simulink model "sanz2016_simu"  (R2023a)
settings: Solver=VariableStepAuto  StartTime=0.0  StopTime=Tsim  RelTol=1e-3
values from neighbouring files (symbols this model uses):
  A = [0 1; -9 3]    [sanz2016_code.m]
  Aw1 = AH_w1    [sanz2016_code.m]
  Aw2 = AH_w2    [sanz2016_code.m]
  B = [0 1]'    [sanz2016_code.m]
  B1w1 = AH_w1*BH_w1*pinv(B)-BH_w1*pinv(B)*A    [sanz2016_code.m]
  B1w2 = AH_w2*BH_w2*pinv(B)-BH_w2*pinv(B)*A    [sanz2016_code.m]
  B2w1 = BH_w1    [sanz2016_code.m]
  B2w2 = BH_w2    [sanz2016_code.m]
  C1 = CH    [sanz2016_code.m]
  C2w1 = CH*BH_w1*pinv(B)    [sanz2016_code.m]
  C2w2 = CH*BH_w2*pinv(B)    [sanz2016_code.m]
  h = 0.5    [sanz2016_code.m]
  K = [-45 -18]    [sanz2016_code.m]
  N = 500    [sanz2016_code.m]
  x0 = [1.5; 1]    [sanz2016_code.m]
undefined symbols (not defined in the file or in its folder): Ad, Bd, Cd, Dd, KSoma, Q, tal
settings Model: Creator=Vasco  LastModifiedBy=Vasco
settings DataIOCC: ReturnWorkspaceOutputs=off

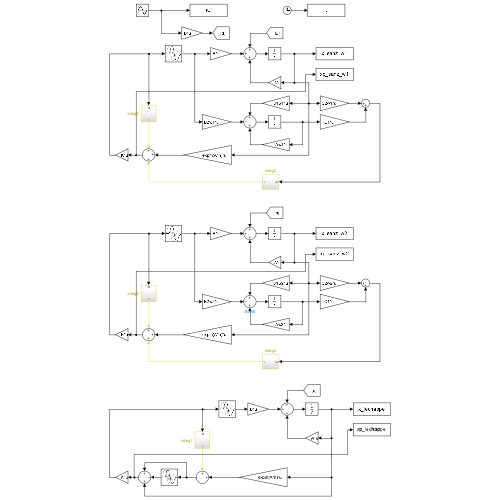
[thumbnail: Simulink's stored preview of the top-level diagram]
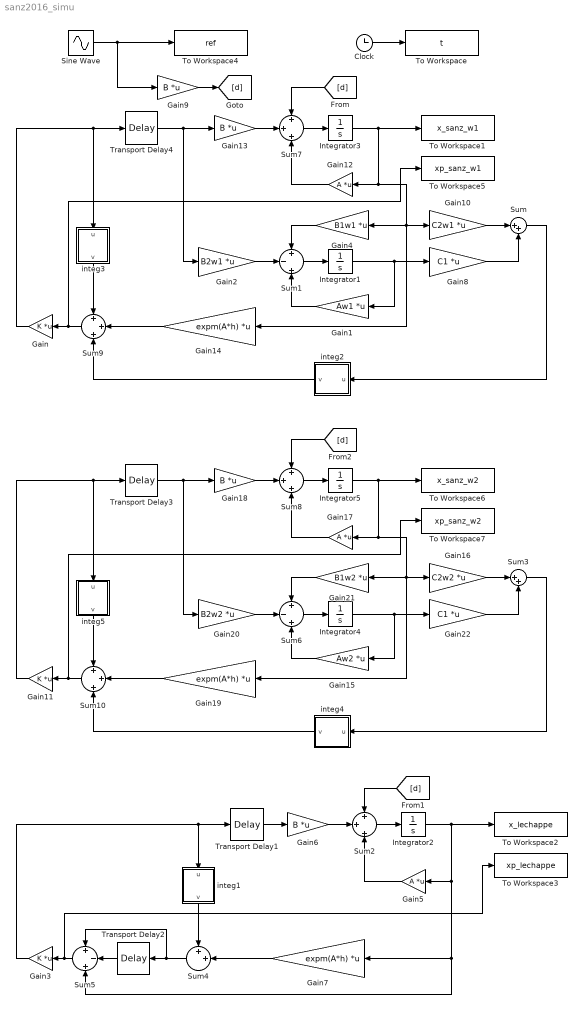
== system sanz2016_simu ==
  Clock : Clock
  Gain : Gain  Gain=K  Multiplication=Matrix(K*u)
  Gain1 : Gain  Gain=Aw1  Multiplication=Matrix(K*u)
  Gain10 : Gain  Gain=C2w1  Multiplication=Matrix(K*u)
  Gain11 : Gain  Gain=K  Multiplication=Matrix(K*u)
  Gain12 : Gain  Gain=A  Multiplication=Matrix(K*u)
  Gain{6,9,13,18} (4 alike) : Gain  Gain=B  Multiplication=Matrix(K*u)
  Gain14 : Gain  Gain=expm(A*h)  Multiplication=Matrix(K*u)
  Gain15 : Gain  Gain=Aw2  Multiplication=Matrix(K*u)
  Gain16 : Gain  Gain=C2w2  Multiplication=Matrix(K*u)
  Gain17 : Gain  Gain=A  Multiplication=Matrix(K*u)
  Gain19 : Gain  Gain=expm(A*h)  Multiplication=Matrix(K*u)
  Gain2 : Gain  Gain=B2w1  Multiplication=Matrix(K*u)
  Gain20 : Gain  Gain=B2w2  Multiplication=Matrix(K*u)
  Gain21 : Gain  Gain=B1w2  Multiplication=Matrix(K*u)
  Gain22 : Gain  Gain=C1  Multiplication=Matrix(K*u)
  Gain3 : Gain  Gain=K  Multiplication=Matrix(K*u)
  Gain4 : Gain  Gain=B1w1  Multiplication=Matrix(K*u)
  Gain5 : Gain  Gain=A  Multiplication=Matrix(K*u)
  Gain7 : Gain  Gain=expm(A*h)  Multiplication=Matrix(K*u)
  Gain8 : Gain  Gain=C1  Multiplication=Matrix(K*u)
  Integrator1 : Integrator
  Integrator2 : Integrator  InitialCondition=x0
  Integrator3 : Integrator  InitialCondition=x0
  Integrator4 : Integrator
  Integrator5 : Integrator  InitialCondition=x0
  Sine Wave : Sin  Amplitude=3  Frequency=0.5  SampleTime=0
  Sum : Sum  Inputs=|++
  Sum1 : Sum  Inputs=+|-|+
  Sum{2,7..10} (5 alike) : Sum  Inputs=+|+|+
  Sum3 : Sum  Inputs=|++
  Sum4 : Sum  Inputs=++|
  Sum5 : Sum  Inputs=+|-|+
  Sum6 : Sum  Inputs=+|-|+
  To Workspace : ToWorkspace  VariableName=t  SampleTime=-1
  To Workspace1 : ToWorkspace  VariableName=x_sanz_w1  SampleTime=-1
  To Workspace2 : ToWorkspace  VariableName=x_lechappe  SampleTime=-1
  To Workspace3 : ToWorkspace  VariableName=xp_lechappe  SampleTime=-1
  To Workspace4 : ToWorkspace  VariableName=ref  SampleTime=-1
  To Workspace5 : ToWorkspace  VariableName=xp_sanz_w1  SampleTime=-1
  To Workspace6 : ToWorkspace  VariableName=x_sanz_w2  SampleTime=-1
  To Workspace7 : ToWorkspace  VariableName=xp_sanz_w2  SampleTime=-1
  Transport Delay{1..4} (4 alike) : TransportDelay  DelayTime=h
  integ1 : Subsystem
  integ2 : Subsystem
  integ3 : Subsystem
  integ4 : Subsystem
  integ5 : Subsystem
  wires:
  Clock/1 -> To Workspace/1
  integ3/1(v) -> Sum9/1
  Gain13/1 -> Sum7/2
  Gain12/1 -> Sum7/3
  Sum7/1 -> Integrator3/1
  Transport Delay4/1 -> Gain13/1, Gain2/1
  Gain14/1 -> Sum9/2
  Gain5/1 -> Sum2/3
  integ1/1(v) -> Sum4/1
  Sum2/1 -> Integrator2/1
  Gain7/1 -> Sum4/2
  Gain6/1 -> Sum2/2
  Transport Delay1/1 -> Gain6/1
  Sum5/1 -> Gain3/1, To Workspace3/1
  Sum4/1 -> Transport Delay2/1, Sum5/1
  Transport Delay2/1 -> Sum5/2
  Sine Wave/1 -> Gain9/1, To Workspace4/1
  Sum9/1 -> To Workspace5/1, Gain/1
  Gain3/1 -> integ1/1(u), Transport Delay1/1
  Gain/1 -> Transport Delay4/1, integ3/1(u)
  Integrator2/1 -> Sum5/3, Gain7/1, Gain5/1, To Workspace2/1
  Gain2/1 -> Sum1/2
  Gain4/1 -> Sum1/1
  Gain1/1 -> Sum1/3
  Integrator1/1 -> Gain8/1, Gain1/1
  Integrator3/1 -> Gain10/1, Gain4/1, Gain14/1, Gain12/1, To Workspace1/1
  Sum1/1 -> Integrator1/1
  Gain10/1 -> Sum/1
  Gain8/1 -> Sum/2
  Sum/1 -> integ2/1(u)
  integ2/1(v) -> Sum9/3
  Gain9/1 -> [d]
  [d] -> Sum7/1
  [d] -> Sum2/1
  integ4/1(v) -> Sum10/3
  Gain16/1 -> Sum3/1
  Gain21/1 -> Sum6/1
  Gain15/1 -> Sum6/3
  Gain11/1 -> Transport Delay3/1, integ5/1(u)
  Sum10/1 -> To Workspace7/1, Gain11/1
  Gain18/1 -> Sum8/2
  Gain17/1 -> Sum8/3
  Integrator4/1 -> Gain22/1, Gain15/1
  Integrator5/1 -> Gain16/1, Gain21/1, Gain19/1, Gain17/1, To Workspace6/1
  Gain22/1 -> Sum3/2
  Gain19/1 -> Sum10/2
  Sum8/1 -> Integrator5/1
  integ5/1(v) -> Sum10/1
  Sum6/1 -> Integrator4/1
  Transport Delay3/1 -> Gain18/1, Gain20/1
  Sum3/1 -> integ4/1(u)
  Gain20/1 -> Sum6/2
  [d] -> Sum8/1

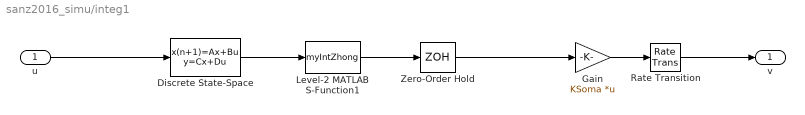
== system sanz2016_simu/integ1 ==
  u : Inport
  Discrete State-Space : DiscreteStateSpace  A=Ad  B=Bd  C=Cd  D=Dd  SampleTime=tal
  Gain : Gain  Gain=KSoma  Multiplication=Matrix(K*u)
  Level-2 MATLAB S-Function1 : M-S-Function  FunctionName=myIntZhong  Parameters=tal,A,B,Q,N
  Rate Transition : RateTransition
  Zero-Order Hold : ZeroOrderHold  SampleTime=tal
  v : Outport  VectorParamsAs1DForOutWhenUnconnected=off
  wires:
  Rate Transition/1 -> v/1
  u/1 -> Discrete State-Space/1
  Gain/1 -> Rate Transition/1
  Zero-Order Hold/1 -> Gain/1
  Discrete State-Space/1 -> Level-2 MATLAB S-Function1/1
  Level-2 MATLAB S-Function1/1 -> Zero-Order Hold/1

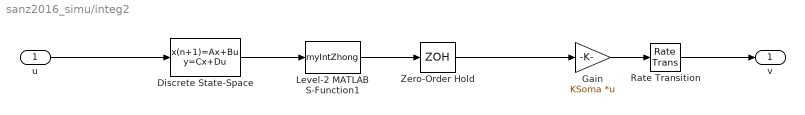
== system sanz2016_simu/integ2 ==
  u : Inport
  Discrete State-Space : DiscreteStateSpace  A=Ad  B=Bd  C=Cd  D=Dd  SampleTime=tal
  Gain : Gain  Gain=KSoma  Multiplication=Matrix(K*u)
  Level-2 MATLAB S-Function1 : M-S-Function  FunctionName=myIntZhong  Parameters=tal,A,B,Q,N
  Rate Transition : RateTransition
  Zero-Order Hold : ZeroOrderHold  SampleTime=tal
  v : Outport  VectorParamsAs1DForOutWhenUnconnected=off
  wires:
  Rate Transition/1 -> v/1
  u/1 -> Discrete State-Space/1
  Gain/1 -> Rate Transition/1
  Zero-Order Hold/1 -> Gain/1
  Discrete State-Space/1 -> Level-2 MATLAB S-Function1/1
  Level-2 MATLAB S-Function1/1 -> Zero-Order Hold/1

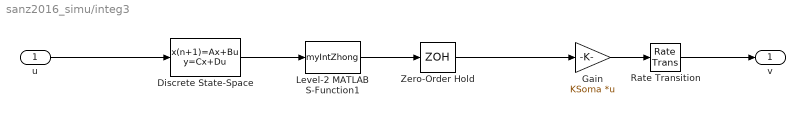
== system sanz2016_simu/integ3 ==
  u : Inport
  Discrete State-Space : DiscreteStateSpace  A=Ad  B=Bd  C=Cd  D=Dd  SampleTime=tal
  Gain : Gain  Gain=KSoma  Multiplication=Matrix(K*u)
  Level-2 MATLAB S-Function1 : M-S-Function  FunctionName=myIntZhong  Parameters=tal,A,B,Q,N
  Rate Transition : RateTransition
  Zero-Order Hold : ZeroOrderHold  SampleTime=tal
  v : Outport  VectorParamsAs1DForOutWhenUnconnected=off
  wires:
  Rate Transition/1 -> v/1
  u/1 -> Discrete State-Space/1
  Gain/1 -> Rate Transition/1
  Zero-Order Hold/1 -> Gain/1
  Discrete State-Space/1 -> Level-2 MATLAB S-Function1/1
  Level-2 MATLAB S-Function1/1 -> Zero-Order Hold/1

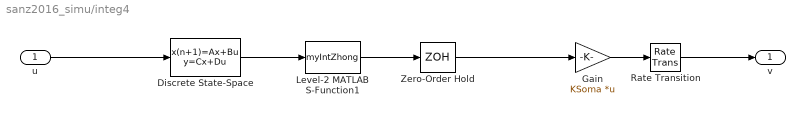
== system sanz2016_simu/integ4 ==
  u : Inport
  Discrete State-Space : DiscreteStateSpace  A=Ad  B=Bd  C=Cd  D=Dd  SampleTime=tal
  Gain : Gain  Gain=KSoma  Multiplication=Matrix(K*u)
  Level-2 MATLAB S-Function1 : M-S-Function  FunctionName=myIntZhong  Parameters=tal,A,B,Q,N
  Rate Transition : RateTransition
  Zero-Order Hold : ZeroOrderHold  SampleTime=tal
  v : Outport  VectorParamsAs1DForOutWhenUnconnected=off
  wires:
  Rate Transition/1 -> v/1
  u/1 -> Discrete State-Space/1
  Gain/1 -> Rate Transition/1
  Zero-Order Hold/1 -> Gain/1
  Discrete State-Space/1 -> Level-2 MATLAB S-Function1/1
  Level-2 MATLAB S-Function1/1 -> Zero-Order Hold/1

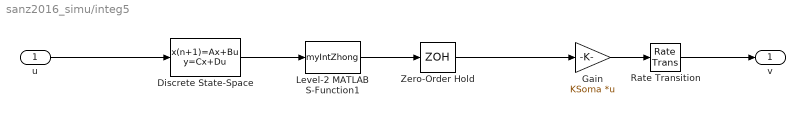
== system sanz2016_simu/integ5 ==
  u : Inport
  Discrete State-Space : DiscreteStateSpace  A=Ad  B=Bd  C=Cd  D=Dd  SampleTime=tal
  Gain : Gain  Gain=KSoma  Multiplication=Matrix(K*u)
  Level-2 MATLAB S-Function1 : M-S-Function  FunctionName=myIntZhong  Parameters=tal,A,B,Q,N
  Rate Transition : RateTransition
  Zero-Order Hold : ZeroOrderHold  SampleTime=tal
  v : Outport  VectorParamsAs1DForOutWhenUnconnected=off
  wires:
  Rate Transition/1 -> v/1
  u/1 -> Discrete State-Space/1
  Gain/1 -> Rate Transition/1
  Zero-Order Hold/1 -> Gain/1
  Discrete State-Space/1 -> Level-2 MATLAB S-Function1/1
  Level-2 MATLAB S-Function1/1 -> Zero-Order Hold/1
